simulink subsystem "x6_dof_robot"  (R2023a)
settings: Solver=VariableStepAuto  StartTime=0.0  StopTime=10.0  RelTol=1e-3
undefined symbols (not defined in the file or in its folder): forward_kinematics
settings Model: Creator=motya  LastModifiedBy=motya

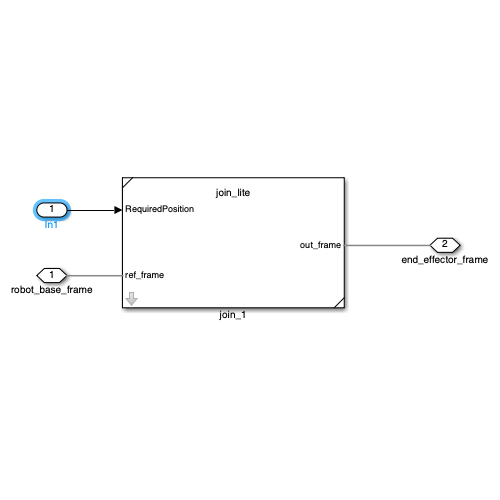
[thumbnail: Simulink's stored preview of the top-level diagram]
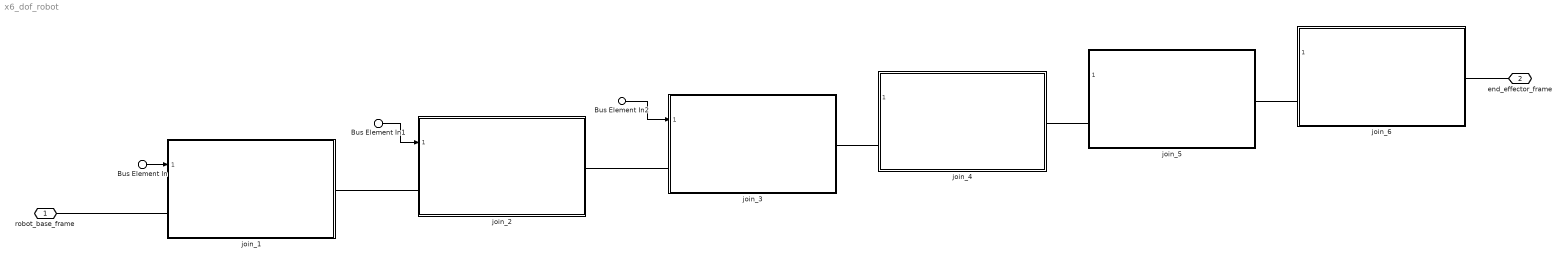
== system x6_dof_robot ==
  Bus Element In : Inport  PortName=positions  Element=join_1_pos
  Bus Element In1 : Inport  PortName=positions  Element=join_2_pos
  Bus Element In2 : Inport  PortName=positions  Element=join_3_pos
  join_1 : Subsystem  ReferencedSubsystem=join_lite  up_limit=180  low_limit=-180  out_frame_rot="forward_kinematics.zero_rot_between_frames(0,  0)"  out_frame_shift="forward_kinematics.zero_shift_between_frames(0,  0)"
  join_2 : Subsystem  ReferencedSubsystem=join_lite  up_limit=180  low_limit=-180  out_frame_rot="forward_kinematics.zero_rot_between_frames(0,  1)"  out_frame_shift="forward_kinematics.zero_shift_between_frames(0,  1)"
  join_3 : Subsystem  ReferencedSubsystem=join_lite  up_limit=180  low_limit=-180  out_frame_rot="forward_kinematics.zero_rot_between_frames(1,  2)"  out_frame_shift="forward_kinematics.zero_shift_between_frames(1,  2)"
  join_4 : Subsystem  ReferencedSubsystem=join_lite  up_limit=180  low_limit=-180  out_frame_rot="forward_kinematics.zero_rot_between_frames(2,  3)"  out_frame_shift="forward_kinematics.zero_shift_between_frames(2,  3)"
  join_5 : Subsystem  ReferencedSubsystem=join_lite  up_limit=180  low_limit=-180  out_frame_rot="forward_kinematics.zero_rot_between_frames(3,  4)"  out_frame_shift=forward_kinematics.zero_shift_between_frames(3, 4)
  join_6 : Subsystem  ReferencedSubsystem=join_lite  up_limit=180  low_limit=-180  out_frame_rot="forward_kinematics.zero_rot_between_frames(4,  5)"  out_frame_shift="forward_kinematics.zero_shift_between_frames(4,  5)"
  robot_base_frame : PMIOPort  Side=Left
  end_effector_frame : PMIOPort  Port=2  Side=Right
  wires:
  Bus Element In/1 -> join_1/1
  Bus Element In1/1 -> join_2/1
  Bus Element In2/1 -> join_3/1
  connections:
  join_1/LConn1 -- robot_base_frame/RConn1
  join_2/LConn1 -- join_1/RConn1
  join_3/LConn1 -- join_2/RConn1
  join_5/LConn1 -- join_4/RConn1
  join_3/RConn1 -- join_4/LConn1
  end_effector_frame/RConn1 -- join_6/RConn1
  join_6/LConn1 -- join_5/RConn1
